simulink model "ANS_GFM_short_term"  (R2021b)
settings: Solver=FixedStepAuto  StartTime=0.0  StopTime=5  FixedStep=Ts  MaxStep=1e-5  RelTol=1e-3
values from neighbouring files (symbols this model uses):
  angle_load = angle(LF.bus(ind_l).Vbus)*180/pi    [init_ANS_GFM_long_term.m]    (also in init_ANS_GFM_short_term.m)
  angleV_LF = Vangle_init/180*pi    [init_ANS_GFM_long_term.m]    (also in init_ANS_GFM_short_term.m)
  awu = 1    [init_ANS_GFM_long_term.m]    (also in init_ANS_GFM_short_term.m)
  C_dc = 1/(Xcdc_pu_or*Zbase_dc_new*100*pi)    [init_ANS_GFM_long_term.m]    (also in init_ANS_GFM_short_term.m)
  C_f = 1/(Xcf_pu_or*Zbase_new*100*pi)    (= 0.013712)    [init_ANS_GFM_long_term.m]    (also in init_ANS_GFM_short_term.m = 0.0141333333333)
  control = 3    [init_ANS_GFM_long_term.m]    (also in init_ANS_GFM_short_term.m = 1)
  D_p = (1/(m_p*w_b))    (= 5209935.26289)    [init_ANS_GFM_long_term.m]    (also in init_ANS_GFM_short_term.m = 5370022.73304)
  Egrid_tmp = 1.054080675694902*400e3    (= 421632.270278)    [init_ANS_GFM_long_term.m]    (also in init_ANS_GFM_short_term.m)
  epsi = 1e-4    (= 0.0001)    [init_ANS_GFM_long_term.m]    (also in init_ANS_GFM_short_term.m)
  eta = m_p*V_m^2    [init_ANS_GFM_long_term.m]    (also in init_ANS_GFM_short_term.m)
  gamma = 2.3    [init_ANS_GFM_long_term.m]    (also in init_ANS_GFM_short_term.m)
  I0_init = [I0_init_a, I0_init_b, I0_init_c]    [init_ANS_GFM_long_term.m]    (also in init_ANS_GFM_short_term.m)
  I_bc = S_bc / (V_bc*sqrt(3))    [init_ANS_GFM_long_term.m]    (also in init_ANS_GFM_short_term.m)
  I_d_int_init = (U_d_int + I_q_int*L_f*w_b - V_d_int - I_d_int*R_f*0)    [init_ANS_GFM_long_term.m]    (also in init_ANS_GFM_short_term.m)
  I_init = [I_init_a, I_init_b, I_init_c]    [init_ANS_GFM_long_term.m]    (also in init_ANS_GFM_short_term.m)
  i_ll = -1.15*(S_bc/Vdc_n)-i_loss_dc    [init_ANS_GFM_long_term.m]    (also in init_ANS_GFM_short_term.m)
  I_max_sat_pu = 1.0 * I_bc *sqrt(2)    [init_ANS_GFM_long_term.m]    (also in init_ANS_GFM_short_term.m)
  I_q_int_init = (U_q_int - I_d_int*L_f*w_b - V_q_int - I_q_int*R_f*0)    [init_ANS_GFM_long_term.m]    (also in init_ANS_GFM_short_term.m)
  i_ul = 1.15*(S_bc/Vdc_n)+i_loss_dc    [init_ANS_GFM_long_term.m]    (also in init_ANS_GFM_short_term.m)
  idppu = 0.95    [init_ANS_GFM_long_term.m]    (also in init_ANS_GFM_short_term.m = 0.92)
  init_dP = -inv(A_pm)*B_pm*dP    [init_ANS_GFM_long_term.m]    (also in init_ANS_GFM_short_term.m)
  init_pm = -inv(A_pm)*B_pm*P_aft    [init_ANS_GFM_long_term.m]    (also in init_ANS_GFM_short_term.m)
  init_tau = -inv(A_tau)*B_tau*idc    [init_ANS_GFM_long_term.m]    (also in init_ANS_GFM_short_term.m)
  J = D_p*tau_f    (= 104198.705258)    [init_ANS_GFM_long_term.m]    (also in init_ANS_GFM_short_term.m = 107400.454661)
  k_dc = eta_1/(Vdc_n*m_p)    [init_ANS_GFM_long_term.m]    (also in init_ANS_GFM_short_term.m)
  K_p = (1/Vdc_n)    [init_ANS_GFM_long_term.m]    (also in init_ANS_GFM_short_term.m)
  K_r = 1/R_dc    [init_ANS_GFM_long_term.m]    (also in init_ANS_GFM_short_term.m)
  Kff_i = 1    [init_ANS_GFM_long_term.m]    (also in init_ANS_GFM_short_term.m)
  Kff_v = 1    [init_ANS_GFM_long_term.m]    (also in init_ANS_GFM_short_term.m)
  Ki_i = (1/n)*1.19    (= 0.0520711785298)    [init_ANS_GFM_long_term.m]    (also in init_ANS_GFM_short_term.m = 0.0505188679245)
  Ki_pll = 4255.3    [init_ANS_GFM_long_term.m]    (also in init_ANS_GFM_short_term.m)
  Ki_v = (n)*1.161022    (= 26.5332227733)    [init_ANS_GFM_long_term.m]    (also in init_ANS_GFM_short_term.m = 27.3485182222)
  ki_v_ac = 2*0.25    (= 0.5)    [init_ANS_GFM_long_term.m]    (also in init_ANS_GFM_short_term.m)
  Kp_i = 0.738891/n    (= 0.032331869895)    [init_ANS_GFM_long_term.m]    (also in init_ANS_GFM_short_term.m = 0.0313680141509)
  Kp_pll = 92    [init_ANS_GFM_long_term.m]    (also in init_ANS_GFM_short_term.m)
  Kp_v = 0.52*n    (= 11.8837333333)    [init_ANS_GFM_long_term.m]    (also in init_ANS_GFM_short_term.m = 12.2488888889)
  kp_v_ac = 0.001    [init_ANS_GFM_long_term.m]    (also in init_ANS_GFM_short_term.m)
  Kpl = 5.0    (= 5)    [init_ANS_GFM_long_term.m]    (also in init_ANS_GFM_short_term.m)
  L1 = cf/sqrt(1+RX^2)*(400e3)^2/Skss/(100*pi)    [init_ANS_GFM_long_term.m]    (also in init_ANS_GFM_short_term.m)
  L_f = Xlf_pu_or*Zbase_new/100/pi    (= 4.37572928821e-06)    [init_ANS_GFM_long_term.m]    (also in init_ANS_GFM_short_term.m = 4.24528301887e-06)
  Lf = 1e6/100/pi    (= 3183.09886184)    [init_ANS_GFM_long_term.m]    (also in init_ANS_GFM_short_term.m = 0.0636619772368)
  m_p = (2*pi*0.5)/(S_bc)    (= 6.10967066042e-10)    [init_ANS_GFM_long_term.m]    (also in init_ANS_GFM_short_term.m = 5.92753330866e-10)
  n = 1/Zb    (= 22.8533333333)    [init_ANS_GFM_long_term.m]    (also in init_ANS_GFM_short_term.m = 23.5555555556)
  P_LF_si = P_LF*S_b    [init_ANS_GFM_long_term.m]    (also in init_ANS_GFM_short_term.m)
  ps = 4440e6/S_bc    (= 0.863477246208)    [init_ANS_GFM_long_term.m]    (also in init_ANS_GFM_short_term.m = 0.837735849057)
  Q_LF_si = Q_LF*S_b    [init_ANS_GFM_long_term.m]    (also in init_ANS_GFM_short_term.m)
  qs = Q_LF*S_b/S_bc    [init_ANS_GFM_long_term.m]    (also in init_ANS_GFM_short_term.m)
  R1 = RX*cf/sqrt(1+RX^2)*(400e3)^2/Skss    [init_ANS_GFM_long_term.m]    (also in init_ANS_GFM_short_term.m)
  R_dc = Rdc_pu_or*Zbase_dc_new    [init_ANS_GFM_long_term.m]    (also in init_ANS_GFM_short_term.m)
  R_f = Rf_pu_or*Zbase_new    (= 2.18786464411e-05)    [init_ANS_GFM_long_term.m]    (also in init_ANS_GFM_short_term.m = 2.12264150943e-05)
  Rf = 1e6    (= 1000000)    [init_ANS_GFM_long_term.m]    (also in init_ANS_GFM_short_term.m = 20)
  S_bc = 5142e6    (= 5142000000)    [init_ANS_GFM_long_term.m]    (also in init_ANS_GFM_short_term.m = 5300000000)
  sat_select = 3    [init_ANS_GFM_long_term.m]    (also in init_ANS_GFM_short_term.m)
  SECM = 3    [init_ANS_GFM_long_term.m]    (also in init_ANS_GFM_short_term.m = 1)
  share_i_load = 1.0    (= 1)    [init_ANS_GFM_long_term.m]    (also in init_ANS_GFM_short_term.m)
  T_en = -0.5    [init_ANS_GFM_long_term.m]    (also in init_ANS_GFM_short_term.m)
  T_off = T_on + 0.1    (= 0.2)    [init_ANS_GFM_long_term.m]    (also in init_ANS_GFM_short_term.m)
  T_on = 0.1    [init_ANS_GFM_long_term.m]    (also in init_ANS_GFM_short_term.m)
  Ts = 2e-6    (= 2e-06)    [init_ANS_GFM_long_term.m]    (also in init_ANS_GFM_short_term.m = 1e-06)
  U_init = [Umag_init_a, Umag_init_b, Umag_init_c]    [init_ANS_GFM_long_term.m]    (also in init_ANS_GFM_short_term.m)
  Uangle_init = angle(V_LF_VSC)*180/pi    [init_ANS_GFM_long_term.m]    (also in init_ANS_GFM_short_term.m)
  Umag_init = abs(V_LF_VSC)*V_bc*sqrt(2/3)    [init_ANS_GFM_long_term.m]    (also in init_ANS_GFM_short_term.m)
  V1_rms = 15e3    (= 15000)    [init_ANS_GFM_long_term.m]    (also in init_ANS_GFM_short_term.m)
  V_d_int = abs(V_LF)*V_bc*sqrt(2/3)    [init_ANS_GFM_long_term.m]    (also in init_ANS_GFM_short_term.m)
  V_d_int_init = (I_d_int + V_q_int*C_f*w_b - I0_d_int)    [init_ANS_GFM_long_term.m]    (also in init_ANS_GFM_short_term.m)
  V_init = [V_init_a, V_init_b, V_init_c]    [init_ANS_GFM_long_term.m]    (also in init_ANS_GFM_short_term.m)
  V_m = sqrt(2/3)*V_bc    [init_ANS_GFM_long_term.m]    (also in init_ANS_GFM_short_term.m)
  V_q_int_init = (I_q_int - V_d_int*C_f*w_b - I0_q_int)    [init_ANS_GFM_long_term.m]    (also in init_ANS_GFM_short_term.m)
  Vdc_n = 3*V_m    [init_ANS_GFM_long_term.m]    (also in init_ANS_GFM_short_term.m)
  Vref = V_LF_mag*V_m    [init_ANS_GFM_long_term.m]    (also in init_ANS_GFM_short_term.m)
  w_b = 2*pi*f_b    (= 314.159265359)    [init_ANS_GFM_long_term.m]    (also in init_ANS_GFM_short_term.m)
  w_f = 2*pi*5    (= 31.4159265359)    [init_ANS_GFM_long_term.m]    (also in init_ANS_GFM_short_term.m)
  Zbase_new = V1_rms^2/S_bc    (= 0.0437572928821)    [init_ANS_GFM_long_term.m]    (also in init_ANS_GFM_short_term.m = 0.0424528301887)
undefined symbols (not defined in the file or in its folder): A_pm, A_tau, B_pm, B_tau, C_pm, C_tau, D_pm, D_tau, find_system, idq0_init, Pm, sm_init, v_d, v_q, Ve
libraries: spsBreakerLib x270, spsGroundLib x21, spsThreePhaseSeriesRLCBranchLib x12, spsabctodq0Lib x11, simulink x9, spsEdgeDetectorLib x8, spsThreePhaseVIMeasurementLib x7, spsLoadFlowBusLib x7, spsSeriesRLCBranchLib x6, spsControlledVoltageSourceLib x6, spsCurrentMeasurementLib x6, spsVoltageMeasurementLib x6
(part 1 of 7)
settings Model: SimulationMode=rapid-accelerator  Creator=Liemann  LastModifiedBy=liemann
settings SolverCC: AlgebraicLoopSolver=TrustRegion
settings DataIOCC: InitialState=xInit  SaveFinalState=on  SaveOperatingPoint=on  SaveOutput=off  SignalLogging=off  DSMLogging=off  SaveTime=off  ReturnWorkspaceOutputs=off
settings OptimizationCC: AccelVerboseBuild=on
settings DebuggingCC: UnconnectedInputMsg=none  UnconnectedOutputMsg=none  UnconnectedLineMsg=none  SFMachineParentedDataDiag=warning  ArithmeticOperatorsInVariantConditions=warning
settings SFSimCC: SimUseLocalCustomCode=off  CustomCodeUndefinedFunction=UseInterfaceOnly
settings RTWCC: RTWUseLocalCustomCode=off  Toolchain=MinGW64 | gmake (64-bit Windows)  BuildConfiguration=Faster Runs
settings CodeAppCC: StateflowObjectComments=on
settings SimscapeCC: SimscapeNormalizeSystem=off

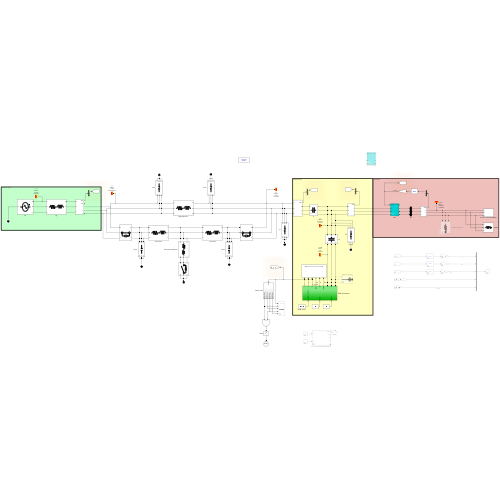
[thumbnail: Simulink's stored preview of the top-level diagram]
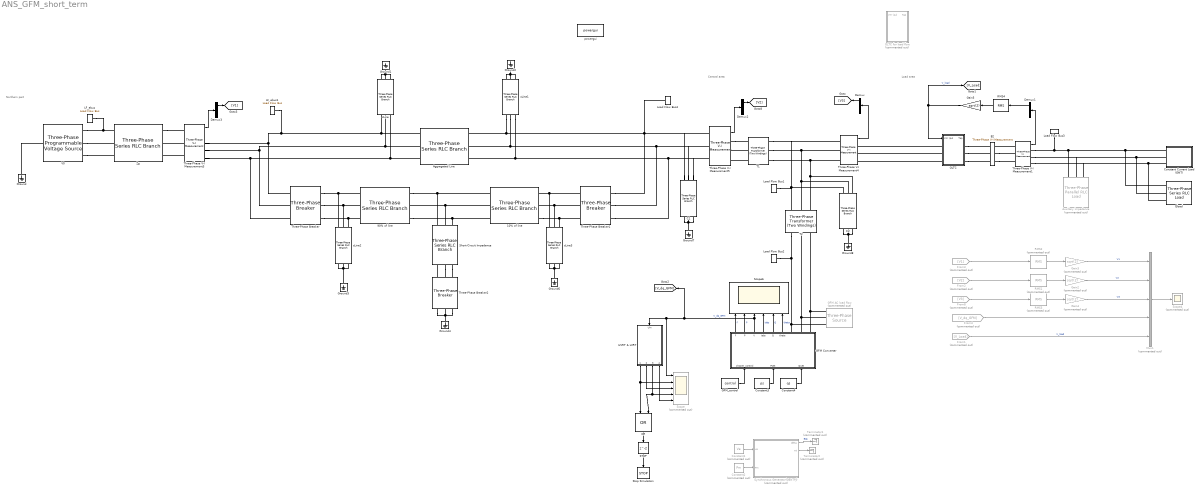
== system ANS_GFM_short_term ==
  note: Load area
  note: Northern part
  note: Central area
  10% of line : spsThreePhaseSeriesRLCBranchLib/Three-Phase Series RLC Branch  LConnTagsString=A|B|C  RConnTagsString=A|B|C  BranchType=RL  Resistance=9.6*0.1  Inductance=80/(2*pi*50)*0.1  Capacitance=1.0  Measurements=None
  "90% of line " : spsThreePhaseSeriesRLCBranchLib/Three-Phase Series RLC Branch  LConnTagsString=A|B|C  RConnTagsString=A|B|C  BranchType=RL  Resistance=9.6*0.9  Inductance=80/(2*pi*50)*0.9  Capacitance=1.0  Measurements=None
  Aggregated Line : spsThreePhaseSeriesRLCBranchLib/Three-Phase Series RLC Branch  LConnTagsString=A|B|C  RConnTagsString=A|B|C  BranchType=RL  Resistance=3.140255  Inductance=17.48548/(2*pi*50)  Capacitance=1.0  Measurements=None
  Auxillary impedance : spsThreePhaseParallelRLCLoadLib/Three-Phase Parallel RLC Load  Commented=on  LConnTagsString=A|B|C  Configuration=Y (grounded)  NominalVoltage=110e3  Vabc=[1e3 1e3 1e3]  Vabcp=[1e3 1e3 1e3]  NominalFrequency=50  UnbalancedPower=off  ActivePower=1000  InductivePower=0  CapacitivePower=0  Pabc=[10e3 9e3 11e3]  QLabc=[100 90 110]  QCabc=[100 90 110]  Pabcp=[10e3 9e3 11e3]  QLabcp=[100 90 110]  QCabcp=[100 90 110]  Measurements=None  LoadType=constant Z
  B2 : spsThreePhaseVIMeasurementLib/Three-Phase V-I Measurement  VoltageMeasurement=phase-to-ground  SetLabelV=on  LabelV=VabcOLTC  Vpu=on  VpuLL=off  CurrentMeasurement=no  SetLabelI=on  LabelI=IabcB2  Ipu=on  Pbase=pnom  Vbase=20e3  OutputType=Complex  PhasorSimulation=off  PSBequivalent=0
  C1 : spsThreePhaseSeriesRLCBranchLib/Three-Phase Series RLC Branch  LConnTagsString=A|B|C  RConnTagsString=A|B|C  BranchType=C  Resistance=120e3^2/1000000e9/10  Inductance=120e3^2/10000000e9/(2*pi*50)  Capacitance=600e6/(400e3^2*100*pi)  Measurements=None
  C2 : spsThreePhaseSeriesRLCBranchLib/Three-Phase Series RLC Branch  LConnTagsString=A|B|C  RConnTagsString=A|B|C  BranchType=C  Resistance=120e3^2/1000000e9/10  Inductance=120e3^2/10000000e9/(2*pi*50)  Capacitance=850e6/(130e3^2*100*pi)  Measurements=None
  Constant Current Load (EMT) : Subsystem  mask{Pload=7580e6*share_i_load, Urms=20e3, angle=angle_load, Kp=Kp_pll, Ki=Ki_pll}
      mask prompts: Pload "Active Power (W)"; Urms "RMS phase-to-phase Voltage (V)"; angle "Uangle Init (deg)"; Kp "Proportional Gain Kp"; Ki "Integral Gain Ki"
      mask init:
      | Ipeakphase = sqrt(2)*Pload/(sqrt(3)*Urms);
      mask DialogControl Container2 Prompt: Control Parameters
  Constant1 : Constant  Commented=on  Value=Ve
  Constant2 : Constant  Commented=on  Value=Pm
  Constant3 : Constant  Value=ps
  Constant4 : Constant  Value=qs
  Demux{,1..3} (4 alike) : Demux  Outputs=3
  From1 : From  Commented=on  GotoTag=V_Load
  From2 : From  Commented=on  GotoTag=V2
  From3 : From  Commented=on  GotoTag=V1
  From4 : From  Commented=on  GotoTag=V_dq_GFM
  From8 : From  Commented=on  GotoTag=V3
  GFM AC load flow : spsThreePhaseSourceLib/Three-Phase Source  Commented=on  InternalConnection=Yg  VoltagePhases=off  Voltage=V1_rms  PhaseAngle=0  Voltage_phases=[25e3 25e3 25e3]/sqrt(3)  PhaseAngles_phases=[0 -120 +120]  Frequency=50  NonIdealSource=off  SpecifyImpedance=off  Resistance=0  Inductance=0  ShortCircuitLevel=100e6  BaseVoltage=Un  XRratio=7  BusType=PV  Pref=S_bc*ps  Qref=Q_ref  Prefabc=[10e3, 10e3, 10e3]  Qrefabc=[0, 0, 0]  Qmin=-sqrt(S_bc^2-(S_bc*ps)^2)+V1_rms^2/(1/(C_f*100*pi))  Qmax=sqrt(S_bc^2-(S_bc*ps)^2)+V1_rms^2/(1/(C_f*100*pi))
  GFM Converter : Subsystem
  GFM_control : Constant  Value=control
  Gain2 : Gain  Commented=on  Gain=sqrt(2)
  Gain3 : Gain  Commented=on  Gain=sqrt(2)
  Gain4 : Gain  Commented=on  Gain=sqrt(2)
  Gain5 : Gain  Gain=sqrt(2)
  Ground{,1..4,6..8} (8 alike) : spsGroundLib/Ground  LConnTagsString=a
  HVRT & LVRT : Subsystem
  LF_ebus : spsLoadFlowBusLib/Load Flow Bus  LConnTagsString=a  Phases=single  Connectors=on one side  ID=v_0  Vbase=400e3  Vref=Egrid_tmp/400e3  Vangle=phase_tmp  VLF=1.054  VLFb=1  VLFc=1  angleLF=18.84  angleLFb=0  angleLFc=0
      settings: SourceProductBaseCode=PS
  LF_ebus1 : spsLoadFlowBusLib/Load Flow Bus  LConnTagsString=a  Phases=single  Connectors=on one side  ID=v_1  Vbase=400e3  Vref=1.036  Vangle=phase_tmp  VLF=1.036  VLFb=1  VLFc=1  angleLF=-0.0002492  angleLFb=0  angleLFc=0
      settings: SourceProductBaseCode=PS
  Load Flow Bus1 : spsLoadFlowBusLib/Load Flow Bus  LConnTagsString=a  Phases=single  Connectors=on one side  ID=v_3  Vbase=130e3  Vref=1  Vangle=0  VLF=0.9731  VLFb=1  VLFc=1  angleLF=-18.5  angleLFb=0  angleLFc=0
      settings: SourceProductBaseCode=PS
  Load Flow Bus2 : spsLoadFlowBusLib/Load Flow Bus  LConnTagsString=a  Phases=single  Connectors=on one side  ID=v_GFM  Vbase=15e3  Vref=1  Vangle=0  VLF=1  VLFb=1  VLFc=1  angleLF=-10.7  angleLFb=0  angleLFc=0
      settings: SourceProductBaseCode=PS
  Load Flow Bus3 : spsLoadFlowBusLib/Load Flow Bus  LConnTagsString=a  Phases=single  Connectors=on one side  ID=v_load  Vbase=20e3  Vref=1  Vangle=0  VLF=0.9903  VLFb=1  VLFc=1  angleLF=4.982  angleLFb=0  angleLFc=0
      settings: SourceProductBaseCode=PS
  Load Flow Bus4 : spsLoadFlowBusLib/Load Flow Bus  LConnTagsString=a  Phases=single  Connectors=on one side  ID=v_2  Vbase=400e3  Vref=1  Vangle=0  VLF=1.027  VLFb=1  VLFc=1  angleLF=-15.73  angleLFb=0  angleLFc=0
      settings: SourceProductBaseCode=PS
  Mux1 : Mux  Commented=on  Inputs=5
  OLTC : Subsystem  LoadFcn=find_system(gcs,'FollowLinks', 'on', 'LookUnderMasks', 'all');  mask(Three-Phase OLTC Regulating Transformer Yg/(D1) -17 positions){ShowParam=OLTC and Voltage Regulator parameters, NominalParameters=[8000e6  50], Winding1=[130e3 0.0 0.11], Winding2=[20e3 0 0.0], RXpuTaps=[0.0 0.0], RXmag=[5000 5000], SetSaturation=off, SaturationCurrentFlux=[0 0; 0.002 1.0; 0.006 1.12; 0.009 1.15; 0.015 1.17; 0.03 1.19; 0.05 1.20; 0.08 1.21; 1.0 1.302], DeltaU=0.01, InitialTap=6, TapSelectionTime=0.0001, TransferTime=0.0, TransR=[1e8 1e-6], RegulatorOn=on, Regulator=[1.  0.02 10]}
      mask prompts: ShowParam "Show"; NominalParameters "Nominal power and frequency [ Pnom(VA)  Fnom(Hz)]:"; Winding1 "Winding 1 (Yg) [V2(Vrms Ph Ph) R1(pu)  X1(pu) ]:"; Winding2 "Winding 2 (D1) [V2(Vrms Ph Ph) R2(pu)  X2(pu) ]"; RXpuTaps "Tapped regulation winding [Rt(pu)  Xt(pu)]"; RXmag "Magnetization branch  [Rm(pu) Lm(pu)]"; SetSaturation "Simulate saturation:"; SaturationCurrentFlux "Saturation characteristic [i1 phi; i2 phi2; ....] (pu)"; DeltaU "Voltage step DeltaU per tap (pu)"; InitialTap "Initial tap position"; TapSelectionTime "Tap selection time (s) (typical 3-10s)"; TransferTime "Tap transition time (s) (typical 40-60 ms)"; TransR "Transfer and Switch resistances  [Ohm Ohm]"; RegulatorOn "Voltage regulator"; Regulator "Voltage regulator [ Vref(pu) DeadBand(pu)  Delay(s)]"
      mask help:
      | The On Load Tap Changer (OLTC) uses a tapped winding (regulation winding) in series with winding 1(Yg) to vary the U1 voltage in 16 DeltaU steps from tap -8 to +8 (17 positions). Tap position 0 corresponds to nominal voltage ratio.
      | The transformer voltage ratio U2/U1 (in pu) is given by:
      |                 U2/U1= 1/ (1+TapPosition*DeltaU)
      | where:
      |               -8<=TapPosition<=+8
      | In automatic mode, ('Voltage regulator'  'on'), the signal applied at the 'Vm' input is monitored and the voltage regulator asks for a tap change if:
      |                  abs(Vm-Vref)>DeadBand/2  during a time  t > Delay.
      mask init:
      | % Below is the only line to modify
      | % to change number of taps
      | NumberOfTaps=20; 
      | 
      | if ~(abs(InitialTap)<=NumberOfTaps & (ceil(InitialTap)-InitialTap)==0)
      |    message = sprintf('The initial tap number must be an integer comprised between % d and %d',-NumberOfTaps,NumberOfTaps);
      |    Erreur.message = message;
      |    Erreur.identifier = 'SimscapePowerSystemsST:OLTCTransformer:ParameterError';
      |    powericon('psberror',Erreur.message,Erreur.identifier,'NoUiwait');
      | end
      | 
      | Rtransfer = TransR(1);
      | Rswitch = TransR(2);
      | Rsnubber = 1e7;
      | Pnom=NominalParameters(1)/3;
      | Fnom=NominalParameters(2);
      | Vnom1= Winding1(1);
      | Vnom2=Winding2(1)/sqrt(3);
      | VnomTaps=Vnom2*DeltaU*(NumberOfTaps);
      | Rpu1= Winding1(2);
      | Rpu2=Winding2(2);
      | RpuTaps=RXpuTaps(1);
      | Xpu1= Winding1(3);
      | Xpu2=Winding2(3);
      | XpuTaps=RXpuTaps(2);
      | Rm=RXmag(1);
      | Lm=RXmag(2);
      | 
      | % Saturation
      | if SetSaturation==1
      | 	set_param([gcb,'/TransformerA'],'SetSaturation','on');
      |     set_param([gcb,'/TransformerB'],'SetSaturation','on');
      |     set_param([gcb,'/TransformerC'],'SetSaturation','on');
      | else
      | 	set_param([gcb,'/TransformerA'],'SetSaturation','off');
      |     set_param([gcb,'/TransformerB'],'SetSaturation','off');
      |     set_param([gcb,'/TransformerC'],'SetSaturation','off');
      | end
      | RegulatorVref=Regulator(1);
      | RegulatorDeadBand=Regulator(2);
      | RegulatorDelay=Regulator(3);
      mask TypeOptions ShowParam: Transformer parameters | OLTC and Voltage Regulator parameters
      mask Callback ShowParam:
      | tempMaskVis=get_param(gcb,'MaskVisibilities');
      | if strcmp(get_param(gcb,'ShowParam'),'Transformer parameters')
      | 	tempMaskVis{2}='on'; tempMaskVis{3}='on'; tempMaskVis{4}='on'; tempMaskVis{5}='on';
      | 	tempMaskVis{6}='on'; tempMaskVis{7}='on';
      | 	if strcmp(get_param(gcb,'SetSaturation'),'on')
      | 		tempMaskVis{8}='on';
      | 	end
      | 	tempMaskVis{9}='off'; tempMaskVis{10}='off'; tempMaskVis{11}='off'; tempMaskVis{12}='off';
      | 	tempMaskVis{13}='off'; tempMaskVis{14}='off'; tempMaskVis{15}='off';
      | 	set_param(gcb,'MaskVisibilities',tempMaskVis);
      | else
      | 	tempMaskVis{2}='off'; tempMaskVis{3}='off'; tempMaskVis{4}='off'; tempMaskVis{5}='off';
      | 	tempMaskVis{6}='off'; tempMaskVis{7}='off'; tempMaskVis{8}='off';
      | 	tempMaskVis{9}='on'; tempMaskVis{10}='on'; tempMaskVis{11}='on'; tempMaskVis{12}='on';
      | 	tempMaskVis{13}='on'; tempMaskVis{14}='on';
      | 	if strcmp(get_param(gcb,'RegulatorOn'),'on')
      | 		tempMaskVis{15}='on';
      | 	end
      | 	set_param(gcb,'MaskVisibilities',tempMaskVis);
      | end
      mask Callback SetSaturation:
      | tempMaskVis=get_param(gcb,'MaskVisibilities');
      | if strcmp(get_param(gcb,'SetSaturation'),'on') & strcmp(get_param(gcb,'ShowParam'),'Transformer parameters')
      | 	tempMaskVis{8}='on';
      | 	set_param(gcb,'MaskVisibilities',tempMaskVis);
      | else
      | 	tempMaskVis{8}='off';
      | 	set_param(gcb,'MaskVisibilities',tempMaskVis);
      | end
      mask TypeOptions RegulatorOn: off | on
      mask Callback RegulatorOn:
      | tempMaskVis=get_param(gcb,'MaskVisibilities');
      | if strcmp(get_param(gcb,'RegulatorOn'),'on') & ~strcmp(get_param(gcb,'ShowParam'),'Transformer parameters')
      | 	tempMaskVis{15}='on';
      | 	set_param(gcb,'MaskVisibilities',tempMaskVis);
      | else
      | 	tempMaskVis{15}='off';
      | 	set_param(gcb,'MaskVisibilities',tempMaskVis);
      | end
  OLTC for load flow : Subsystem  Commented=on  LoadFcn=find_system(gcs,'FollowLinks', 'on', 'LookUnderMasks', 'all');  mask(Three-Phase OLTC Regulating Transformer Yg/(D1) -17 positions){ShowParam=OLTC and Voltage Regulator parameters, NominalParameters=[8000e6  50], Winding1=[130e3 0.0 0.11], Winding2=[20e3 0 0], RXpuTaps=[0.0 0.0], RXmag=[5000 5000], SetSaturation=off, SaturationCurrentFlux=[0 0; 0.002 1.0; 0.006 1.12; 0.009 1.15; 0.015 1.17; 0.03 1.19; 0.05 1.20; 0.08 1.21; 1.0 1.302], DeltaU=0.01, InitialTap=6, TapSelectionTime=0.0001, TransferTime=0.0, TransR=[1e8 1e-5], RegulatorOn=on, Regulator=[1.  0.02 10]}
      mask prompts: ShowParam "Show"; NominalParameters "Nominal power and frequency [ Pnom(VA)  Fnom(Hz)]:"; Winding1 "Winding 1 (Yg) [V2(Vrms Ph Ph) R1(pu)  X1(pu) ]:"; Winding2 "Winding 2 (D1) [V2(Vrms Ph Ph) R2(pu)  X2(pu) ]"; RXpuTaps "Tapped regulation winding [Rt(pu)  Xt(pu)]"; RXmag "Magnetization branch  [Rm(pu) Lm(pu)]"; SetSaturation "Simulate saturation:"; SaturationCurrentFlux "Saturation characteristic [i1 phi; i2 phi2; ....] (pu)"; DeltaU "Voltage step DeltaU per tap (pu)"; InitialTap "Initial tap position"; TapSelectionTime "Tap selection time (s) (typical 3-10s)"; TransferTime "Tap transition time (s) (typical 40-60 ms)"; TransR "Transfer and Switch resistances  [Ohm Ohm]"; RegulatorOn "Voltage regulator"; Regulator "Voltage regulator [ Vref(pu) DeadBand(pu)  Delay(s)]"
      mask help:
      | The On Load Tap Changer (OLTC) uses a tapped winding (regulation winding) in series with winding 1(Yg) to vary the U1 voltage in 16 DeltaU steps from tap -8 to +8 (17 positions). Tap position 0 corresponds to nominal voltage ratio.
      | The transformer voltage ratio U2/U1 (in pu) is given by:
      |                 U2/U1= 1/ (1+TapPosition*DeltaU)
      | where:
      |               -8<=TapPosition<=+8
      | In automatic mode, ('Voltage regulator'  'on'), the signal applied at the 'Vm' input is monitored and the voltage regulator asks for a tap change if:
      |                  abs(Vm-Vref)>DeadBand/2  during a time  t > Delay.
      mask init: same as ANS_GFM_short_term/OLTC
      mask TypeOptions ShowParam: Transformer parameters | OLTC and Voltage Regulator parameters
      mask Callback ShowParam:
      | tempMaskVis=get_param(gcb,'MaskVisibilities');
      | if strcmp(get_param(gcb,'ShowParam'),'Transformer parameters')
      | 	tempMaskVis{2}='on'; tempMaskVis{3}='on'; tempMaskVis{4}='on'; tempMaskVis{5}='on';
      | 	tempMaskVis{6}='on'; tempMaskVis{7}='on';
      | 	if strcmp(get_param(gcb,'SetSaturation'),'on')
      | 		tempMaskVis{8}='on';
      | 	end
      | 	tempMaskVis{9}='off'; tempMaskVis{10}='off'; tempMaskVis{11}='off'; tempMaskVis{12}='off';
      | 	tempMaskVis{13}='off'; tempMaskVis{14}='off'; tempMaskVis{15}='off';
      | 	set_param(gcb,'MaskVisibilities',tempMaskVis);
      | else
      | 	tempMaskVis{2}='off'; tempMaskVis{3}='off'; tempMaskVis{4}='off'; tempMaskVis{5}='off';
      | 	tempMaskVis{6}='off'; tempMaskVis{7}='off'; tempMaskVis{8}='off';
      | 	tempMaskVis{9}='on'; tempMaskVis{10}='on'; tempMaskVis{11}='on'; tempMaskVis{12}='on';
      | 	tempMaskVis{13}='on'; tempMaskVis{14}='on';
      | 	if strcmp(get_param(gcb,'RegulatorOn'),'on')
      | 		tempMaskVis{15}='on';
      | 	end
      | 	set_param(gcb,'MaskVisibilities',tempMaskVis);
      | end
      mask Callback SetSaturation:
      | tempMaskVis=get_param(gcb,'MaskVisibilities');
      | if strcmp(get_param(gcb,'SetSaturation'),'on') & strcmp(get_param(gcb,'ShowParam'),'Transformer parameters')
      | 	tempMaskVis{8}='on';
      | 	set_param(gcb,'MaskVisibilities',tempMaskVis);
      | else
      | 	tempMaskVis{8}='off';
      | 	set_param(gcb,'MaskVisibilities',tempMaskVis);
      | end
      mask TypeOptions RegulatorOn: off | on
      mask Callback RegulatorOn:
      | tempMaskVis=get_param(gcb,'MaskVisibilities');
      | if strcmp(get_param(gcb,'RegulatorOn'),'on') & ~strcmp(get_param(gcb,'ShowParam'),'Transformer parameters')
      | 	tempMaskVis{15}='on';
      | 	set_param(gcb,'MaskVisibilities',tempMaskVis);
      | else
      | 	tempMaskVis{15}='off';
      | 	set_param(gcb,'MaskVisibilities',tempMaskVis);
      | end
  OR : Logic  Operator=OR  IconShape=distinctive  AllPortsSameDT=off  OutDataTypeStr=boolean
  Qload : spsThreePhaseSeriesRLCLoadLib/Three-Phase Series RLC Load  LConnTagsString=A|B|C  Configuration=Y (grounded)  NominalVoltage=20e3  Vabc=[1e3 1e3 1e3]  Vabcp=[1e3 1e3 1e3]  NominalFrequency=50  UnbalancedPower=off  ActivePower=7580e6*(1-share_i_load)  InductivePower=2243700000  CapacitivePower=0  Pabc=[10e3 9e3 11e3]  QLabc=[100 90 110]  QCabc=[100 90 110]  Pabcp=[10e3 9e3 11e3]  QLabcp=[100 90 110]  QCabcp=[100 90 110]  Measurements=None  LoadType=constant Z
  RMS1 : spsRMSLib/RMS  Commented=on  TrueRMS=off  Freq=50  RMSInit=init_v2  Ts=0
  RMS2 : spsRMSLib/RMS  Commented=on  TrueRMS=off  Freq=50  RMSInit=init_v1  Ts=0
  RMS3 : spsRMSLib/RMS  Commented=on  TrueRMS=off  Freq=50  RMSInit=init_v3  Ts=0
  RMS4 : spsRMSLib/RMS  TrueRMS=on  Freq=50  RMSInit=init_vload  Ts=0
  STOP : Delay
  Scope : Scope  Commented=on  NumInputPorts=5
  Scope4 : Scope  Commented=on
  Scope6 : Scope  NumInputPorts=6
  Short-Circuit Impedance : spsThreePhaseSeriesRLCBranchLib/Three-Phase Series RLC Branch  LConnTagsString=A|B|C  RConnTagsString=A|B|C  BranchType=RL  Resistance=Rf  Inductance=Lf  Capacitance=1.0  Measurements=None
  Stop Simulation : Stop
  Synchronous Generator(GENTPJ) : Subsystem  Commented=on  mask{Sbase=5300e6, Sbase_grid=8000e6, Urms=15e3, cosphi=0.83, pgen=4400e6, H=6, D=0, Ra=0, Xl=0.15, Xd=2.2, Xq=2.0, Xds=0.3, Xqs=0.4, Xdss=0.2, Xqss=0.2, Td0s=7, Tq0s=1.5, Td0ss=0.05, Tq0ss=0.05, S10=0.1, S12=0.3, init=sm_init}
      mask prompts: Sbase "Base apparent power SM (W)"; Sbase_grid "Base apparent power grid (W)"; Urms "Base RMS line-line voltage (V)"; cosphi "Power Factor"; pgen "Active power operation point (W)"; H "Inertia (H)"; D "Damping (D)"; Ra "Ra (pu)"; Xl "Xl (pu)"; Xd "Xd  (pu)"; Xq "Xq (pu)"; Xds "Xd' (pu)"; Xqs "Xq' (pu)"; Xdss "Xd'' (pu)"; Xqss "Xq'' (pu)"; Td0s "Td0' (s)"; Tq0s "Tq0' (s)"; Td0ss "Td0'' (s)"; Tq0ss "Tq0'' (s)"; S10 "S10 (pu)"; S12 "S12 (pu)"; init "[Eangle Uini Phiinit Ed' Eq' Ed'' Eq'']"
      mask init:
      | delta0_init= init(1);
      | Urmsinit = init(2);
      | phiinit = init(3);
      | 
      | eds = init(4);
      | eqs = init(5);
      | edss = init(6);
      | eqss = init(7);
      | 
      | 
      | Pbase = Sbase*cosphi;
      | 
      | Qmax = Pbase * sqrt(1 / (cosphi^2) - 1);
      | Qmin = -Qmax;
      | 
      | q = log(S12/S10)/log(1.2);
      mask DialogControl DescGroupVar Prompt: Base parameters
      mask DialogControl Container3 Prompt: Mechanical Parameters
      mask DialogControl Container4 Prompt: Electrical parameters
      mask DialogControl Container6 Prompt: Saturation paramers (exp.)
      mask DialogControl Container7 Prompt: Initialisation
  T1 : spsThreePhaseTransformerTwoWindingsLib/Three-Phase Transformer (Two Windings)  Winding1Connection=Y  Winding2Connection=Y  CoreType=Three single-phase transformers  SetSaturation=off  Hysteresis=off  DataFile='hysteresis'  SetInitialFlux=off  Measurements=None  UNITS=pu  NominalPower=[8000e6 , 50]  Winding1=[400e3*1.05, 0, 1e-5]  Winding2=[130e3, 1e-4*0, 0.12]  Rm=50000  Lm=50000  L0=0.5  Saturation=[ 0,0 ; 0.0024,1.2 ; 1.0,1.52 ]  InitialFluxes=[ 0.8 , -0.8 , 0.7 ]  BreakLoop=off  DiscreteSolver=Trapezoidal iterative  DataType=off  TransfoNumber=1
  T2 : spsThreePhaseTransformerTwoWindingsLib/Three-Phase Transformer (Two Windings)  Winding1Connection=Y  Winding2Connection=Y  CoreType=Three single-phase transformers  SetSaturation=off  Hysteresis=off  DataFile='hysteresis'  SetInitialFlux=off  Measurements=None  UNITS=pu  NominalPower=[5300e6, 50 ]  Winding1=[15e3, 0, 1e-5]  Winding2=[130e3*1.05, 1e-4*0, 0.15]  Rm=50000  Lm=50000  L0=1.5  Saturation=[0 0;0.0008 3.5999;0.33334 4.5602]  InitialFluxes=[2.4 -2.4 2.1]  BreakLoop=off  DiscreteSolver=Trapezoidal iterative  DataType=off  TransfoNumber=1
  Terminator1 : Terminator  Commented=on
  Terminator2 : Terminator  Commented=on
  Three-Phase V-I Measurement1 : spsThreePhaseVIMeasurementLib/Three-Phase V-I Measurement  VoltageMeasurement=phase-to-ground  SetLabelV=off  LabelV=Vabc  Vpu=on  VpuLL=off  CurrentMeasurement=no  SetLabelI=off  LabelI=Iabc  Ipu=off  Pbase=100e6  Vbase=20e3  OutputType=Magnitude  PhasorSimulation=off  PSBequivalent=0
  Three-Phase V-I Measurement3 : spsThreePhaseVIMeasurementLib/Three-Phase V-I Measurement  VoltageMeasurement=phase-to-ground  SetLabelV=off  LabelV=Vabc  Vpu=on  VpuLL=off  CurrentMeasurement=yes  SetLabelI=off  LabelI=Iabc  Ipu=off  Pbase=100e6  Vbase=400e3  OutputType=Magnitude  PhasorSimulation=off  PSBequivalent=0
  Three-Phase V-I Measurement4 : spsThreePhaseVIMeasurementLib/Three-Phase V-I Measurement  VoltageMeasurement=phase-to-ground  SetLabelV=off  LabelV=Vabc  Vpu=on  VpuLL=off  CurrentMeasurement=no  SetLabelI=off  LabelI=Iabc  Ipu=off  Pbase=1000e6  Vbase=130e3  OutputType=Magnitude  PhasorSimulation=off  PSBequivalent=0
  Three-Phase V-I Measurement5 : spsThreePhaseVIMeasurementLib/Three-Phase V-I Measurement  VoltageMeasurement=phase-to-ground  SetLabelV=off  LabelV=Vabc  Vpu=on  VpuLL=off  CurrentMeasurement=no  SetLabelI=off  LabelI=Iabc  Ipu=off  Pbase=1000e6  Vbase=400e3  OutputType=Magnitude  PhasorSimulation=off  PSBequivalent=0
  Three-Phase Breaker : spsThreePhaseBreakerLib/Three-Phase Breaker  InitialState=closed  SwitchA=on  SwitchB=on  SwitchC=on  SwitchTimes=[T_off]  External=off  BreakerResistance=0.001  SnubberResistance=1e9  SnubberCapacitance=inf  Measurements=None
  Three-Phase Breaker1 : spsThreePhaseBreakerLib/Three-Phase Breaker  InitialState=closed  SwitchA=on  SwitchB=on  SwitchC=on  SwitchTimes=[T_off]  External=off  BreakerResistance=0.001  SnubberResistance=1e8  SnubberCapacitance=inf  Measurements=None
  Three-Phase Breaker2 : spsThreePhaseBreakerLib/Three-Phase Breaker  InitialState=open  SwitchA=on  SwitchB=on  SwitchC=on  SwitchTimes=[T_on T_off]  External=off  BreakerResistance=0.001  SnubberResistance=1e9  SnubberCapacitance=inf  Measurements=None
  V0 : spsThreePhaseProgrammableVoltageSourceLib/Three-Phase Programmable Voltage Source  PositiveSequence=[(400000)*1.05408 18.8429 50]  VariationEntity=None  VariationType=Table of time-amplitude pairs  VariationTypeAlt=Step  VariationStep=0.2  VariationRate=10  VariationMagnitude=0.3  VariationFrequency=2  VariationTiming="[5  20]"  VariationPhaseA=off  Amplitudes=[ 1 ]  TimeValues=[0]  HarmonicGeneration=off  HarmonicA=[3 0.2 -25 0]  HarmonicB=[2 0.15 35 2]  Timing="[0.05  3]"  BusType=swing  Pref=0  Qref=0  Qmin=-Inf  Qmax=Inf
  Zg : spsThreePhaseSeriesRLCBranchLib/Three-Phase Series RLC Branch  LConnTagsString=A|B|C  RConnTagsString=A|B|C  BranchType=RL  Resistance=R1  Inductance=L1  Capacitance=1.0  Measurements=None
  cLine : spsThreePhaseSeriesRLCBranchLib/Three-Phase Series RLC Branch  LConnTagsString=A|B|C  RConnTagsString=A|B|C  BranchType=C  Resistance=120e3^2/1000000e9/10  Inductance=120e3^2/10000000e9/(2*pi*50)  Capacitance=19.49005e-6/2  Measurements=None
  cLine1 : spsThreePhaseSeriesRLCBranchLib/Three-Phase Series RLC Branch  LConnTagsString=A|B|C  RConnTagsString=A|B|C  BranchType=C  Resistance=120e3^2/1000000e9/10  Inductance=120e3^2/10000000e9/(2*pi*50)  Capacitance=19.49005e-6/2  Measurements=None
  cLine2 : spsThreePhaseSeriesRLCBranchLib/Three-Phase Series RLC Branch  LConnTagsString=A|B|C  RConnTagsString=A|B|C  BranchType=C  Resistance=120e3^2/1000000e9/10  Inductance=120e3^2/10000000e9/(2*pi*50)  Capacitance=4.77e-6/2  Measurements=None
  cLine3 : spsThreePhaseSeriesRLCBranchLib/Three-Phase Series RLC Branch  LConnTagsString=A|B|C  RConnTagsString=A|B|C  BranchType=C  Resistance=120e3^2/1000000e9/10  Inductance=120e3^2/10000000e9/(2*pi*50)  Capacitance=4.77e-6/2  Measurements=None
  powergui : spspowerguiLib/powergui  Priority=1  SimulationMode=Discrete  SampleTime=Ts  frequency=50  Iterations=50  frequencyindice=50  Pbase=8000e6  ErrMax=1e-8  UnitsV=kV  UnitsW=MW  buscounter=14  FunctionMessages=on  echomessages=on  EnableUseOfTLC=off  CurrentSourceSwitches=off  DisableSnubberDevices=off  DisableRonSwitches=off  DisableVfSwitches=off  DisplayEquations=off  AutomaticDiscreteSolvers=off  SolverType=Tustin/Backward Euler (TBE)  Interpol=off  ExternalGateDelay=off  methode=off  Ts=100  x0status=steady  SPID=on  SwTol=0  HookPort=off  NonlinearTolerance=1e-4  nMaxIteration=100  ContinueOnMaxIteration=off  RestoreLinks=warning  ResistiveCurrentMeasurement=off  Frange=[0:2:500]  Ylog=off  Xlog=on  ShowGrid=off  save=off  variable=ZData  structure=0  ZoomFFT=off  StartTime=0.0  cycles=1  DisplayStyle=1  fundamental=60  FreqAxis=off  MaxFrequency=1000  frequencyindicesteady=1  RmsSteady=2  display=off
  wires:
  From2/1 -> RMS1/1
  Three-Phase V-I Measurement4/1 -> Demux/1
  Demux/1 -> [V3]
  From3/1 -> RMS2/1
  Three-Phase V-I Measurement3/1 -> Demux3/1
  Demux3/1 -> [V1]
  RMS1/1 -> Gain2/1
  RMS2/1 -> Gain3/1
  Gain2/1 -> Mux1/2  "V2"
  Mux1/1 -> Scope4/1
  Gain3/1 -> Mux1/1  "V1"
  Demux1/1 -> RMS4/1
  Three-Phase V-I Measurement1/1 -> Demux1/1
  Three-Phase V-I Measurement5/1 -> Demux2/1
  Demux2/1 -> [V2]
  From8/1 -> RMS3/1
  RMS3/1 -> Gain4/1
  Gain4/1 -> Mux1/3  "V3"
  Constant1/1 -> Synchronous Generator(GENTPJ)/1(ve)
  Constant2/1 -> Synchronous Generator(GENTPJ)/2(Pm)
  Synchronous Generator(GENTPJ)/1(delta) -> Terminator1/1  "Eqs"
  Synchronous Generator(GENTPJ)/2(wt) -> Terminator2/1
  GFM Converter/4(Iabs) -> Scope6/4  "iabs"
  GFM Converter/5(Q) -> Scope6/5  "Q"
  GFM Converter/1(f) -> Scope6/1  "f"
  GFM Converter/2(P) -> Scope6/2  "P"
  GFM Converter/6(theta) -> Scope6/6  "theta"
  From1/1 -> Mux1/5  "V_load"
  GFM_control/1 -> GFM Converter/1(chosen_control)
  GFM Converter/3(V) -> Scope6/3, [V_dq_GFM], Scope/1, HVRT & LVRT/1(Uin)  "V_dq_GFM"
  HVRT & LVRT/1(HVRT-Flag) -> Scope/2, OR/1
  HVRT & LVRT/2(HVRT curve) -> Scope/3
  HVRT & LVRT/3(LVRT-Flag) -> OR/2, Scope/4
  HVRT & LVRT/4(LVRT curve) -> Scope/5
  OR/1 -> STOP/1
  STOP/1 -> Stop Simulation/1
  Constant3/1 -> GFM Converter/2(Pset)
  Constant4/1 -> GFM Converter/3(Qset)
  RMS4/1 -> Gain5/1
  Gain5/1 -> OLTC/1(Vm (pu)), [V_Load]  "V_load"
  From4/1 -> Mux1/4
  connections:
  Ground/LConn1 -- V0/LConn1
  Three-Phase Breaker1/RConn1 -- Load Flow Bus4/LConn1 -- Three-Phase V-I Measurement5/LConn1 -- C1/LConn1 -- Aggregated Line/RConn1 -- cLine1/RConn1
  T1/RConn2 -- Three-Phase V-I Measurement4/LConn2 -- C2/LConn2 -- T2/RConn2
  10% of line/RConn3 -- Three-Phase Breaker1/LConn3 -- cLine3/LConn3
  cLine/LConn1 -- Ground1/LConn1 -- cLine/LConn2 -- cLine/LConn3
  cLine1/LConn2 -- cLine1/LConn3 -- Ground2/LConn1 -- cLine1/LConn1
  cLine2/RConn2 -- cLine2/RConn3 -- Ground3/LConn1 -- cLine2/RConn1
  cLine3/RConn2 -- cLine3/RConn3 -- Ground6/LConn1 -- cLine3/RConn1
  Short-Circuit Impedance/LConn2 -- 10% of line/LConn2 -- "90% of line "/RConn2
  "90% of line "/RConn1 -- 10% of line/LConn1 -- Short-Circuit Impedance/LConn1
  "90% of line "/RConn3 -- 10% of line/LConn3 -- Short-Circuit Impedance/LConn3
  "90% of line "/LConn2 -- Three-Phase Breaker/RConn2 -- cLine2/LConn2
  Three-Phase V-I Measurement3/RConn1 -- LF_ebus1/LConn1 -- Aggregated Line/LConn1 -- cLine/RConn1 -- Three-Phase Breaker/LConn1
  Three-Phase V-I Measurement4/LConn1 -- T1/RConn1 -- Load Flow Bus1/LConn1 -- T2/RConn1 -- C2/LConn1
  cLine3/LConn1 -- Three-Phase Breaker1/LConn1 -- 10% of line/RConn1
  Three-Phase Breaker1/RConn3 -- Three-Phase V-I Measurement5/LConn3 -- C1/LConn3 -- Aggregated Line/RConn3 -- cLine1/RConn3
  cLine3/LConn2 -- Three-Phase Breaker1/LConn2 -- 10% of line/RConn2
  cLine2/LConn1 -- Three-Phase Breaker/RConn1 -- "90% of line "/LConn1
  cLine2/LConn3 -- Three-Phase Breaker/RConn3 -- "90% of line "/LConn3
  B2/RConn2 -- Three-Phase V-I Measurement1/LConn2
  B2/RConn3 -- Three-Phase V-I Measurement1/LConn3
  T1/RConn3 -- Three-Phase V-I Measurement4/LConn3 -- C2/LConn3 -- T2/RConn3
  Qload/LConn2 -- Auxillary impedance/LConn2 -- Three-Phase V-I Measurement1/RConn2 -- Constant Current Load (EMT)/LConn2
  Constant Current Load (EMT)/LConn3 -- Auxillary impedance/LConn3 -- Three-Phase V-I Measurement1/RConn3 -- Qload/LConn3
  Qload/LConn1 -- Load Flow Bus3/LConn1 -- Three-Phase V-I Measurement1/RConn1 -- Auxillary impedance/LConn1 -- Constant Current Load (EMT)/LConn1
  cLine1/RConn2 -- Aggregated Line/RConn2 -- Three-Phase Breaker1/RConn2 -- Three-Phase V-I Measurement5/LConn2 -- C1/LConn2
  Ground7/LConn1 -- C1/RConn1 -- C1/RConn2 -- C1/RConn3
  C2/RConn3 -- C2/RConn1 -- Ground8/LConn1 -- C2/RConn2
  Three-Phase Breaker2/RConn1 -- Short-Circuit Impedance/RConn1
  Short-Circuit Impedance/RConn2 -- Three-Phase Breaker2/RConn2
  Short-Circuit Impedance/RConn3 -- Three-Phase Breaker2/RConn3
  Ground4/LConn1 -- Three-Phase Breaker2/LConn2 -- Three-Phase Breaker2/LConn3 -- Three-Phase Breaker2/LConn1
  V0/RConn1 -- LF_ebus/LConn1 -- Zg/LConn1
  V0/RConn2 -- Zg/LConn2
  V0/RConn3 -- Zg/LConn3
  Zg/RConn1 -- Three-Phase V-I Measurement3/LConn1
  Three-Phase V-I Measurement3/LConn2 -- Zg/RConn2
  Three-Phase V-I Measurement3/LConn3 -- Zg/RConn3
  Aggregated Line/LConn2 -- cLine/RConn2 -- Three-Phase Breaker/LConn2 -- Three-Phase V-I Measurement3/RConn2
  Three-Phase V-I Measurement3/RConn3 -- Aggregated Line/LConn3 -- cLine/RConn3 -- Three-Phase Breaker/LConn3
  Three-Phase V-I Measurement5/RConn1 -- T1/LConn1
  T1/LConn2 -- Three-Phase V-I Measurement5/RConn2
  T1/LConn3 -- Three-Phase V-I Measurement5/RConn3
  OLTC/LConn1 -- Three-Phase V-I Measurement4/RConn1
  OLTC/LConn2 -- Three-Phase V-I Measurement4/RConn2
  OLTC/LConn3 -- Three-Phase V-I Measurement4/RConn3
  OLTC/RConn1 -- B2/LConn1
  OLTC/RConn2 -- B2/LConn2
  OLTC/RConn3 -- B2/LConn3
  Three-Phase V-I Measurement1/LConn1 -- B2/RConn1
  GFM Converter/RConn3 -- GFM AC load flow/RConn3 -- T2/LConn3
  T2/LConn1 -- GFM AC load flow/RConn1 -- GFM Converter/RConn1 -- Load Flow Bus2/LConn1
  GFM Converter/RConn2 -- GFM AC load flow/RConn2 -- T2/LConn2

== system ANS_GFM_short_term/Constant Current Load (EMT) ==
  Aux. Impedance : spsThreePhaseSeriesRLCBranchLib/Three-Phase Series RLC Branch  LConnTagsString=A|B|C  RConnTagsString=A|B|C  BranchType=R  Resistance=Urms^2/Pload/1e-5  Inductance=0.10*(110e3)^2/100e6/(2*pi*50)  Capacitance=1.0  Measurements=None
  Controlled Current Source3 : spsControlledCurrentSourceLib/Controlled Current Source  Initialize=on  Source_Type=AC  Amplitude=Ipeakphase  Phase=angle  Frequency=50  Measurements=None
  Controlled Current Source4 : spsControlledCurrentSourceLib/Controlled Current Source  Initialize=on  Source_Type=AC  Amplitude=Ipeakphase  Phase=angle-120  Frequency=50  Measurements=None
  Controlled Current Source5 : spsControlledCurrentSourceLib/Controlled Current Source  Initialize=on  Source_Type=AC  Amplitude=Ipeakphase  Phase=angle+120  Frequency=50  Measurements=None
  Ground1 : spsGroundLib/Ground  LConnTagsString=a
  Ground3 : spsGroundLib/Ground  LConnTagsString=a
  PLL : Subsystem
  Pload - Load Flow : spsThreePhaseSeriesRLCLoadLib/Three-Phase Series RLC Load  Commented=on  LConnTagsString=A|B|C  Configuration=Y (grounded)  NominalVoltage=(20000)*0.995162  Vabc=[1e3 1e3 1e3]  Vabcp=[1e3 1e3 1e3]  NominalFrequency=50  UnbalancedPower=off  ActivePower=Pload  InductivePower=0  CapacitivePower=0  Pabc=[10e3 9e3 11e3]  QLabc=[100 90 110]  QCabc=[100 90 110]  Pabcp=[10e3 9e3 11e3]  QLabcp=[100 90 110]  QCabcp=[100 90 110]  Measurements=None  LoadType=constant I
  Three-Phase V-I Measurement5 : spsThreePhaseVIMeasurementLib/Three-Phase V-I Measurement  VoltageMeasurement=phase-to-ground  SetLabelV=off  LabelV=Vabc  Vpu=on  VpuLL=off  CurrentMeasurement=no  SetLabelI=off  LabelI=Iabc  Ipu=off  Pbase=Pload  Vbase=Urms  OutputType=Magnitude  PhasorSimulation=off  PSBequivalent=0
  A : PMIOPort  Side=Left
  B : PMIOPort  Port=2  Side=Left
  C : PMIOPort  Port=3  Side=Left
  wires:
  Three-Phase V-I Measurement5/1 -> PLL/1(Vabc)
  PLL/2(Ib) -> Controlled Current Source4/1
  PLL/3(Ic) -> Controlled Current Source5/1
  PLL/1(Ia) -> Controlled Current Source3/1
  connections:
  Aux. Impedance/RConn2 -- Ground1/LConn1 -- Aux. Impedance/RConn3 -- Aux. Impedance/RConn1
  Three-Phase V-I Measurement5/RConn2 -- Pload - Load Flow/LConn2 -- Aux. Impedance/LConn2 -- Controlled Current Source4/LConn1
  Three-Phase V-I Measurement5/RConn3 -- Pload - Load Flow/LConn3 -- Aux. Impedance/LConn3 -- Controlled Current Source5/LConn1
  Three-Phase V-I Measurement5/RConn1 -- Pload - Load Flow/LConn1 -- Aux. Impedance/LConn1 -- Controlled Current Source3/LConn1
  Three-Phase V-I Measurement5/LConn3 -- C/RConn1
  Three-Phase V-I Measurement5/LConn1 -- A/RConn1
  Three-Phase V-I Measurement5/LConn2 -- B/RConn1
  Ground3/LConn1 -- Controlled Current Source3/RConn1 -- Controlled Current Source5/RConn1 -- Controlled Current Source4/RConn1
